simulink model "diagrama1"  (Simulink 9.1)
settings: Solver=ode5  StartTime=0.0  StopTime=4.46  FixedStep=1/64000  RelTol=1e-3
libraries: dspobslib x1, dspsrcs4 x1
settings Model: Creator=Eduardo  LastModifiedBy=erban
settings DataIOCC: SignalLoggingSaveFormat=ModelDataLogs  SaveOutput=off  SaveTime=off  SignalLoggingName=sigsOut
settings OptimizationCC: BlockReduction=off  BooleanDataType=off  ExpressionDepthLimit=2147483647
settings DebuggingCC: SaveWithParameterizedLinksMsg=none  SignalResolutionControl=TryResolveAllWithWarning  MultiTaskDSMMsg=warning  MultiTaskCondExecSysMsg=none  FcnCallInpInsideContextMsg=warning  AllowSymbolicDim=off  StateNameClashWarn=warning
settings HardwareCC: ProdHWDeviceType=Specified  TargetUnknown=on

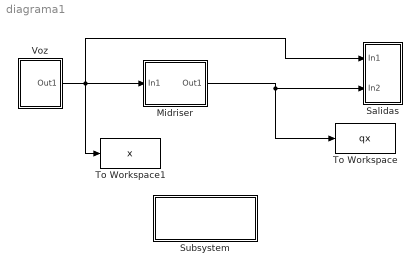
== system diagrama1 ==
  Midriser : Subsystem  mask{L=8, xsc=1}
      mask prompts: L "niveles"
      mask Display: image('.\png\midriser.png');
  Salidas : Subsystem
      mask Display:
      | plot([0, 1], [1, 1]);
      | plot([0, 0], [1, 0.5]);
      | plot([0, 1], [0.5, 0.5]);
      | plot([1, 1], [1, 0.5]);
      | disp('\n\nMulti\nscope');
  Subsystem : Subsystem  mask{L=8, xsc=1}
      mask prompts: L "Niveles :"; xsc "xsc :"
      mask Callback L:
      | L = get_param(gcb, 'L');
      | set_param([bdroot '/Midriser'], 'L',L);
      mask Callback xsc:
      | xsc = get_param(gcb, 'xsc');
      | set_param([bdroot '/Midriser'], 'xsc',xsc);
      mask Display: disp('Parametros del\nsistema');
  To Workspace : ToWorkspace  VariableName=qx  SampleTime=-1
      settings: Save2DSignal=2-D array (concatenate along first dimension)
  To Workspace1 : ToWorkspace  VariableName=x  SampleTime=-1
      settings: Save2DSignal=2-D array (concatenate along first dimension)
  Voz : Subsystem
      mask Display: disp('Voz');
  wires:
  Voz/1(Out1) -> To Workspace1/1, Salidas/1(In1), Midriser/1(In1)
  Midriser/1(Out1) -> Salidas/2(In2), To Workspace/1

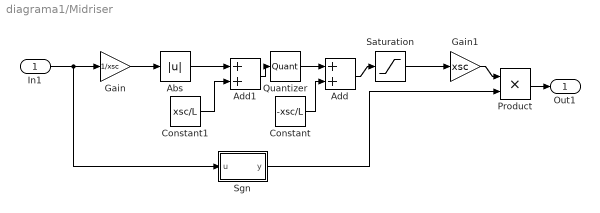
== system diagrama1/Midriser ==
  In1 : Inport
  Abs : Abs
  Add : Sum
  Add1 : Sum
  Constant : Constant  Value=-xsc/L
  Constant1 : Constant  Value=xsc/L
  Gain : Gain  Gain=1/xsc
  Gain1 : Gain  Gain=xsc
  Product : Product
  Quantizer : Quantizer  QuantizationInterval=2*xsc/L
  Saturation : Saturate  UpperLimit=xsc-xsc/L  LowerLimit=-xsc+xsc/L
  Sgn : MATLAB Function  TreatAsAtomicUnit=on
  Out1 : Outport
  wires:
  In1/1 -> Gain/1, Sgn/1(u)
  Product/1 -> Out1/1
  Quantizer/1 -> Add/1
  Sgn/1(y) -> Product/2
  Constant/1 -> Add/2
  Add/1 -> Saturation/1
  Gain1/1 -> Product/1
  Saturation/1 -> Gain1/1
  Add1/1 -> Quantizer/1
  Gain/1 -> Abs/1
  Constant1/1 -> Add1/2
  Abs/1 -> Add1/1

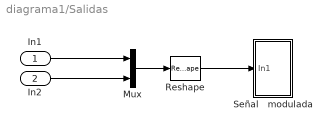
== system diagrama1/Salidas ==
  In1 : Inport
  In2 : Inport  Port=2
  Mux : Mux  Inputs=2
  Reshape : Reshape  OutputDimensionality=Row vector (2-D)
  Señal   modulada : Subsystem
      mask Display:
      | plot([0, 1], [1, 1]);
      | plot([0, 0], [1, 0.5]);
      | plot([0, 1], [0.5, 0.5]);
      | plot([1, 1], [1, 0.5]);
      | disp('\n\nFrame\nscope');
  wires:
  Mux/1 -> Reshape/1
  Reshape/1 -> Señal   modulada/1(In1)
  In1/1 -> Mux/1
  In2/1 -> Mux/2

== system diagrama1/Subsystem ==

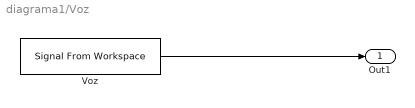
== system diagrama1/Voz ==
  Voz : dspsrcs4/Signal From Workspace  X=audioread('rtve1.wav')  Ts=1/8000  nsamps=1  OutputAfterFinalValue=Setting to zero  ignoreOrWarnInputAndFrameLengths=off  OutputFrames=on
  Out1 : Outport
  wires:
  Voz/1 -> Out1/1

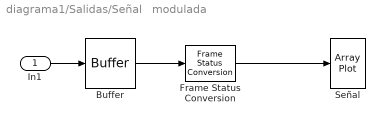
== system diagrama1/Salidas/Señal   modulada ==
  In1 : Inport
  Buffer : Buffer  N=400
  Frame Status Conversion : dspobslib/Frame Status Conversion  growRefPort=off  outframe=Frame-based
      settings: SourceProductBaseCode=DS
  Señal : ArrayPlot
  wires:
  Buffer/1 -> Frame Status Conversion/1
  Frame Status Conversion/1 -> Señal/1
  In1/1 -> Buffer/1

== matlab function Midriser/Sgn ==
  data: u input double; y output double
function y = fcn(u)

if u~=0
    y=sign(u);
else
    y=1;
end
